simulink model "bh_SIM_7dof_car_MODAL_EXCITE"  (R2021a)
settings: Solver=ode15s  StartTime=0.0  StopTime=5  FixedStep=0.0005  RelTol=1e-5
settings Model: Creator=bhorton  LastModifiedBy=bhorton
settings SolverCC: ZeroCrossAlgorithm=Adaptive
settings ExplorerConfigSet: InternalSimMechanicsExplorerSettings="<ExplorerConfiguration><canonicalview>default</canonicalview><AnimationSetting><BasePlaybackSpeed>1.0</BasePlaybackSpeed><PlaybackSpeedFactor>1.0</PlaybackSpeedFactor></AnimationSetting><TilePanel><TileInfo><Tiles Columns=\"2\" Count=\"3\" Rows=\"2\"><Column Weight=\"0.4994\"/><Column Weight=\"0.5006\"/><Row Weight=\"0.4993\"/><Row Weight=\"0.5007\"/><Tile Height=\"1\" Width=\"2\" X=\"0\" Y=\"0\"/><Tile Height=\"1\" Width=\"1\" X=\"0\" Y=\"1\"/><Tile Height=\"1\" Width=\"1\" X=\"1\" Y=\"1\"/></Tiles></TileInfo><SceneInfo><SceneViewer><BGColor><R>0.60000002384185791</R><G>0.60000002384185791</G><B>0.60000002384185791</B></BGColor><Camera><DoPerspective>off</DoPerspective><Position><X>4.52139190602701735</X><Y>2.25786544378109522</Y><Z>2.39499099381060532</Z></Position><Center><X>2.51193884455935335</X><Y>1.32650226914164038</Y><Z>-0.485736887395236794</Z></Center><Up><X>-0.185673330126828295</X><Y>0.96548958646651295</Y><Z>-0.182634259941381938</Z></Up><ViewLimDist>1</ViewLimDist><YLim>1.8643738979882809</YLim><XLim>3.80619953061108962</XLim></Camera></SceneViewer><SceneViewer><BGColor><R>0.60000002384185791</R><G>0.60000002384185791</G><B>0.60000002384185791</B></BGColor><Camera><DoPerspective>off</DoPerspective><Position><X>1.59253986433018846</X><Y>1.4781034625054259</Y><Z>2.45336125750569334</Z></Position><Center><X>1.41562813270534282</X><Y>1.03964723052633357</Y><Z>-0.792996094118513462</Z></Center><Up><X>-0.0228131350943184333</X><Y>0.990908416802929626</Y><Z>-0.132589857742894418</Z></Up><ViewLimDist>1</ViewLimDist><YLim>1.71081238252217549</YLim><XLim>1.71587395761839479</XLim></Camera></SceneViewer><SceneViewer><BGColor><R>0.60000002384185791</R><G>0.60000002384185791</G><B>0.60000002384185791</B></BGColor><Camera><DoPerspective>off</DoPerspective><Position><X>5.22556337212071131</X><Y>1.49802244333944778</Y><Z>-0.435936726178495881</Z></Position><Center><X>1.55561505094653896</X><Y>1.09424096945505833</Y><Z>-0.658674871233751014</Z></Center><Up><X>-0.109797444713875203</X><Y>0.993927323497863835</Y><Z>0.0072798858972461869</Z></Up><ViewLimDist>1</ViewLimDist><YLim>2.32163445502303123</YLim><XLim>2.33537193700541623</XLim></Camera></SceneViewer></SceneInfo></TilePanel><MechEditorPanel><Cameras/><GfxPanelCameraMap/><VideoCreator><PlaybackSpeedRatio>0.25</PlaybackSpeedRatio><FrameRate>30</FrameRate><VideoFormat>MPEG-4</VideoFormat><FrameSize>[800 600]</FrameSize></VideoCreator></MechEditorPanel></ExplorerConfiguration>"

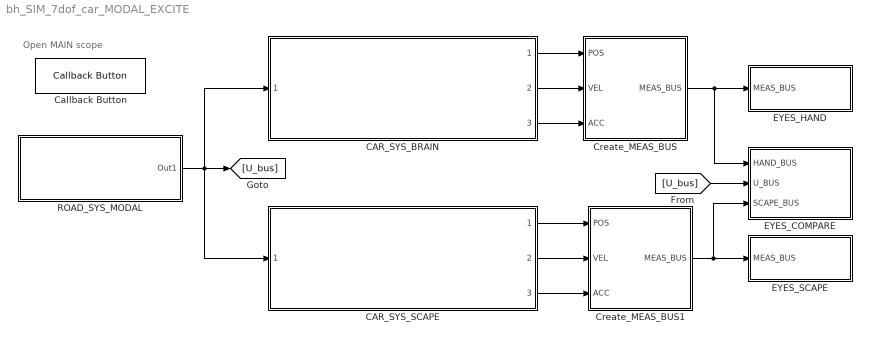
== system bh_SIM_7dof_car_MODAL_EXCITE ==
  note: Open MAIN scope
  CAR_SYS_BRAIN : Subsystem  ReferencedSubsystem=bh_COMPONENT_model_7dof_car_HAND  L_b=OBJ_car_params.L_b  L_f=OBJ_car_params.L_f  L_R=OBJ_car_params.L_R  L_L=OBJ_car_params.L_L  m_c=OBJ_car_params.m_c  I_cZ=OBJ_car_params.I_cZ  I_cX=OBJ_car_params.I_cX  m_bR=OBJ_car_params.m_bR  m_fR=OBJ_car_params.m_fR  m_bL=OBJ_car_params.m_bL  m_fL=OBJ_car_params.m_fL  k_bR=OBJ_car_params.k_bR  k_fR=OBJ_car_params.k_fR  k_bL=OBJ_car_params.k_bL  k_fL=OBJ_car_params.k_fL  k_bRG=OBJ_car_params.k_bRG  k_fRG=OBJ_car_params.k_fRG  k_bLG=OBJ_car_params.k_bLG  k_fLG=OBJ_car_params.k_fLG  c_bR=OBJ_car_params.c_bR  c_fR=OBJ_car_params.c_fR  c_bL=OBJ_car_params.c_bL  c_fL=OBJ_car_params.c_fL  c_bRG=OBJ_car_params.c_bRG  c_fRG=OBJ_car_params.c_fRG  c_bLG=OBJ_car_params.c_bLG  c_fLG=OBJ_car_params.c_fLG  IC_pos=OBJ_car_params.IC_pos  IC_vel=OBJ_car_params.IC_vel
  CAR_SYS_SCAPE : Subsystem  ReferencedSubsystem=bh_COMPONENT_model_7dof_car_SCAPE  L_b=OBJ_car_params.L_b  L_f=OBJ_car_params.L_f  L_R=OBJ_car_params.L_R  L_L=OBJ_car_params.L_L  m_c=OBJ_car_params.m_c  I_cZ=OBJ_car_params.I_cZ  I_cX=OBJ_car_params.I_cX  m_bR=OBJ_car_params.m_bR  m_fR=OBJ_car_params.m_fR  m_bL=OBJ_car_params.m_bL  m_fL=OBJ_car_params.m_fL  k_bR=OBJ_car_params.k_bR  k_fR=OBJ_car_params.k_fR  k_bL=OBJ_car_params.k_bL  k_fL=OBJ_car_params.k_fL  k_bRG=OBJ_car_params.k_bRG  k_fRG=OBJ_car_params.k_fRG  k_bLG=OBJ_car_params.k_bLG  k_fLG=OBJ_car_params.k_fLG  c_bR=OBJ_car_params.c_bR  c_fR=OBJ_car_params.c_fR  c_bL=OBJ_car_params.c_bL  c_fL=OBJ_car_params.c_fL  c_bRG=OBJ_car_params.c_bRG  c_fRG=OBJ_car_params.c_fRG  c_bLG=OBJ_car_params.c_bLG  c_fLG=OBJ_car_params.c_fLG  IC_pos=OBJ_car_params.IC_pos  IC_vel=OBJ_car_params.IC_vel
  Callback Button : CallbackButton  ButtonText=CLICK me to open SCOPE
      settings: ClickFcn=open_system([bdroot,'/EYES_COMPARE/COMPARE_POS'])
  Create_MEAS_BUS : Subsystem
  Create_MEAS_BUS1 : Subsystem
  EYES_COMPARE : Subsystem
  EYES_HAND : Subsystem
  EYES_SCAPE : Subsystem
  ROAD_SYS_MODAL : Subsystem  mask(ROAD_MODAL_EXCITATION){m_AMP=0.03, m_excite_type=bh_excite_mode_ENUM_CLS.MODAL_Y_BOUNCE, f_str=3, m_mode_table={'1', 'BOUNCE','0.9162';  '2', 'ROLL','1.1836';  '3', 'PITCH','1.6742';  '4', 'FRONT_OUT_PHASE','5.6358';  '5', 'FRONT_IN_PHASE','5.6435';  '6', 'BACK_OUT_PHASE','6.2992';  '7', 'BACK_IN_PHASE','6.3188'}}
      mask prompts: m_AMP "Amplitude (m)"; m_excite_type "Excitation Type"; f_str "f (Hz)"; m_mode_table "The Modes (the table is NOT editable)"
      mask help:
      | ATTENTION:
      |
      | The MODAL frequencies are HARD CODED in the function bh_road_modal_callback().
      |
      | So? - So if you configure the car with different parameters(m,ck, etc) then you need to update the above file with your UNdamped modal frequencies.
      mask init:
      | % ATTENTION:
      | %   there is a CALLBACK attached to the "m_excite_type"
      | %   parameter which ENABLES or DISABLES the "f_str"
      | %   parameter.  See the file:
      | %
      | %    --->  bh_road_modal_callback.m
      | 
      | f_hz            = str2num(f_str);
      | excite_type_str = string(m_excite_type);
      | amp_str         = num2str(m_AMP);
      | 
      | str0 = sprintf('%s',excite_type_str);
      | str1 = sprintf('Amp = %s', amp_str);
      | 
      | tf_sine_excite = m_excite_type.isSineMember();
      | 
      | f_hz_modal = 0;
      | 
      | if(tf_sine_excite)
      |     str2 = sprintf('Freq = %d (Hz)',f_hz);
      | else
      |     f_hz_modal = bh_road_modal_callback("GET_FHZ_MODAL", gcb);
      |     str2       = sprintf('Freq = %.4f (Hz)',f_hz_modal);
      | end
      | 
      | str  = char(str0,str1,str2);
      | 
      | bh_road_modal_callback("POPULATE_TABLE", gcb);
      mask Callback m_excite_type: bh_road_modal_callback("M_EXCITE_CBACK", gcb)
      mask TypeOptions f_str: 0 | 1 | 2 | 3 | 5 | 10 | 20 | 50 | 100
      mask DialogControl Container3 Prompt: Edit the following file to define your MODAL frequencies
      mask DialogControl Control2 Prompt: CLICK ME TO EDIT FILE
      mask DialogControl Control2 Callback: bh_road_modal_callback("EDIT_THIS_FILE",gcb)
      mask Display: disp(str)
  wires:
  CAR_SYS_BRAIN/1 -> Create_MEAS_BUS/1(POS)
  CAR_SYS_BRAIN/2 -> Create_MEAS_BUS/2(VEL)
  CAR_SYS_BRAIN/3 -> Create_MEAS_BUS/3(ACC)
  Create_MEAS_BUS/1(MEAS_BUS) -> EYES_COMPARE/1(HAND_BUS), EYES_HAND/1(MEAS_BUS)
  CAR_SYS_SCAPE/1 -> Create_MEAS_BUS1/1(POS)
  CAR_SYS_SCAPE/2 -> Create_MEAS_BUS1/2(VEL)
  CAR_SYS_SCAPE/3 -> Create_MEAS_BUS1/3(ACC)
  Create_MEAS_BUS1/1(MEAS_BUS) -> EYES_COMPARE/3(SCAPE_BUS), EYES_SCAPE/1(MEAS_BUS)
  ROAD_SYS_MODAL/1(Out1) -> [U_bus], CAR_SYS_BRAIN/1, CAR_SYS_SCAPE/1
  [U_bus] -> EYES_COMPARE/2(U_BUS)

== system bh_SIM_7dof_car_MODAL_EXCITE/Create_MEAS_BUS ==
  POS : Inport
  VEL : Inport  Port=2
  ACC : Inport  Port=3
  Bus Creator : BusCreator  Inputs=3
  MEAS_BUS : Outport
  wires:
  POS/1 -> Bus Creator/1  "POS"
  VEL/1 -> Bus Creator/2  "VEL"
  ACC/1 -> Bus Creator/3  "ACC"
  Bus Creator/1 -> MEAS_BUS/1

== system bh_SIM_7dof_car_MODAL_EXCITE/Create_MEAS_BUS1 ==
  POS : Inport
  VEL : Inport  Port=2
  ACC : Inport  Port=3
  Bus Creator : BusCreator  Inputs=3
  MEAS_BUS : Outport
  wires:
  POS/1 -> Bus Creator/1  "POS"
  VEL/1 -> Bus Creator/2  "VEL"
  ACC/1 -> Bus Creator/3  "ACC"
  Bus Creator/1 -> MEAS_BUS/1

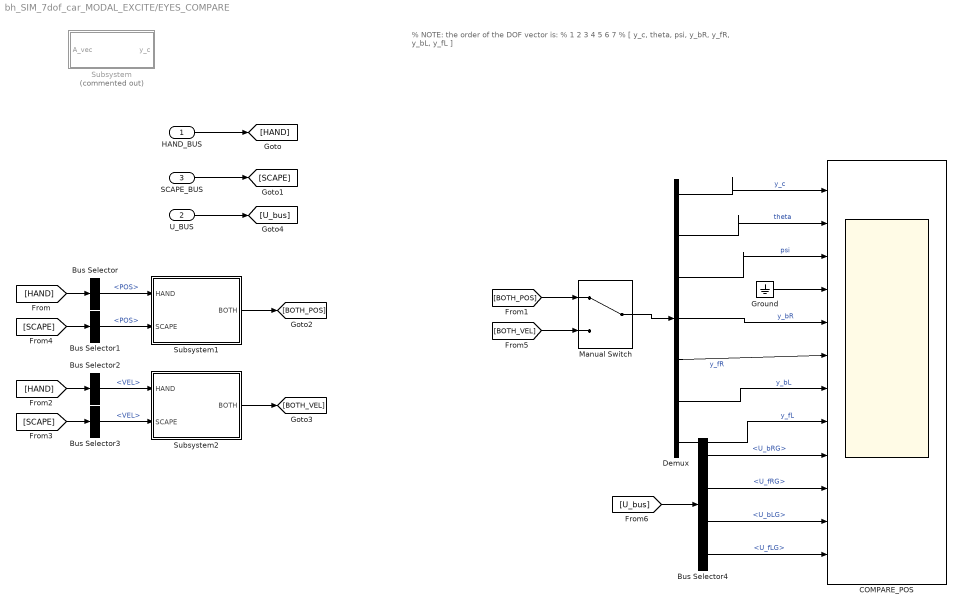
== system bh_SIM_7dof_car_MODAL_EXCITE/EYES_COMPARE ==
  note: % NOTE:  the order of the DOF vector is:
      | %          1      2    3     4     5     6     7
      | %      [ y_c, theta, psi, y_bR, y_fR, y_bL, y_fL ]
  HAND_BUS : Inport
  U_BUS : Inport  Port=2
  SCAPE_BUS : Inport  Port=3
  Bus Selector : BusSelector  OutputSignals=POS
  Bus Selector1 : BusSelector  OutputSignals=POS
  Bus Selector2 : BusSelector  OutputSignals=VEL
  Bus Selector3 : BusSelector  OutputSignals=VEL
  Bus Selector4 : BusSelector  OutputSignals=U_bRG,U_fRG,U_bLG,U_fLG
  COMPARE_POS : Scope  NumInputPorts=12
  Demux : Demux  Outputs=7
  Ground : Ground
  Manual Switch : ManualSwitch
  Subsystem : Subsystem  Commented=on
  Subsystem1 : Subsystem
  Subsystem2 : Subsystem
  wires:
  HAND_BUS/1 -> [HAND]
  Demux/1 -> COMPARE_POS/1  "y_c"
  Demux/2 -> COMPARE_POS/2  "theta"
  Demux/3 -> COMPARE_POS/3  "psi"
  Ground/1 -> COMPARE_POS/4
  Demux/4 -> COMPARE_POS/5  "y_bR"
  Demux/5 -> COMPARE_POS/6  "y_fR"
  Demux/6 -> COMPARE_POS/7  "y_bL"
  Demux/7 -> COMPARE_POS/8  "y_fL"
  SCAPE_BUS/1 -> [SCAPE]
  [HAND] -> Bus Selector/1
  [SCAPE] -> Bus Selector1/1
  Bus Selector/1 -> Subsystem1/1(HAND)  "<POS>"
  Bus Selector1/1 -> Subsystem1/2(SCAPE)  "<POS>"
  Subsystem1/1(BOTH) -> [BOTH_POS]
  [HAND] -> Bus Selector2/1
  Subsystem2/1(BOTH) -> [BOTH_VEL]
  Bus Selector2/1 -> Subsystem2/1(HAND)  "<VEL>"
  Bus Selector3/1 -> Subsystem2/2(SCAPE)  "<VEL>"
  [SCAPE] -> Bus Selector3/1
  Manual Switch/1 -> Demux/1
  [BOTH_VEL] -> Manual Switch/2
  [BOTH_POS] -> Manual Switch/1
  U_BUS/1 -> [U_bus]
  [U_bus] -> Bus Selector4/1
  Bus Selector4/4 -> COMPARE_POS/12  "<U_fLG>"
  Bus Selector4/3 -> COMPARE_POS/11  "<U_bLG>"
  Bus Selector4/2 -> COMPARE_POS/10  "<U_fRG>"
  Bus Selector4/1 -> COMPARE_POS/9  "<U_bRG>"

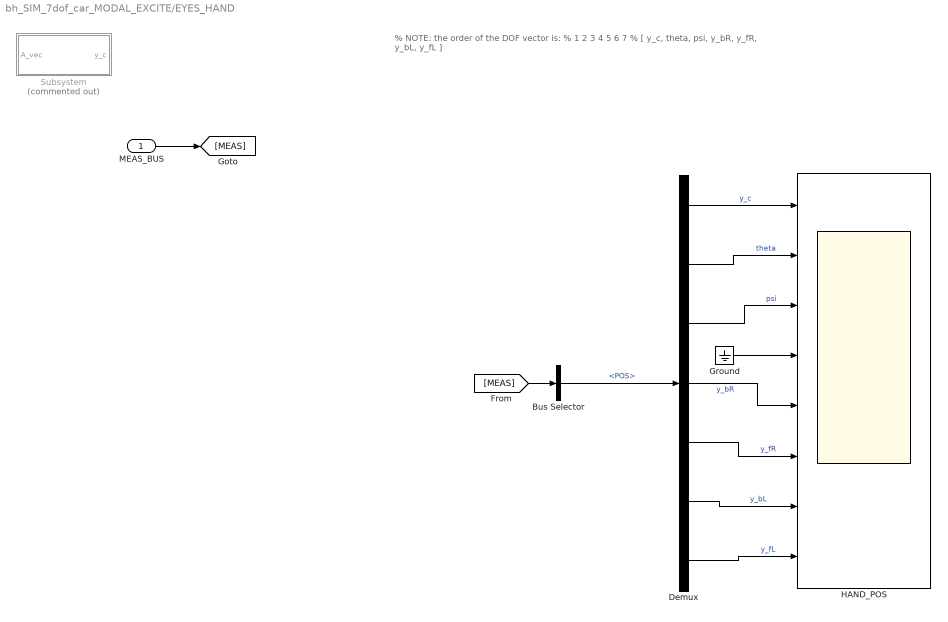
== system bh_SIM_7dof_car_MODAL_EXCITE/EYES_HAND ==
  note: % NOTE:  the order of the DOF vector is:
      | %          1      2    3     4     5     6     7
      | %      [ y_c, theta, psi, y_bR, y_fR, y_bL, y_fL ]
  MEAS_BUS : Inport
  Bus Selector : BusSelector  OutputSignals=POS
  Demux : Demux  Outputs=7
  Ground : Ground
  HAND_POS : Scope  NumInputPorts=8
  Subsystem : Subsystem  Commented=on
  wires:
  MEAS_BUS/1 -> [MEAS]
  Demux/1 -> HAND_POS/1  "y_c"
  Demux/2 -> HAND_POS/2  "theta"
  Demux/3 -> HAND_POS/3  "psi"
  Ground/1 -> HAND_POS/4
  Demux/4 -> HAND_POS/5  "y_bR"
  Demux/5 -> HAND_POS/6  "y_fR"
  Demux/6 -> HAND_POS/7  "y_bL"
  Demux/7 -> HAND_POS/8  "y_fL"
  [MEAS] -> Bus Selector/1
  Bus Selector/1 -> Demux/1  "<POS>"

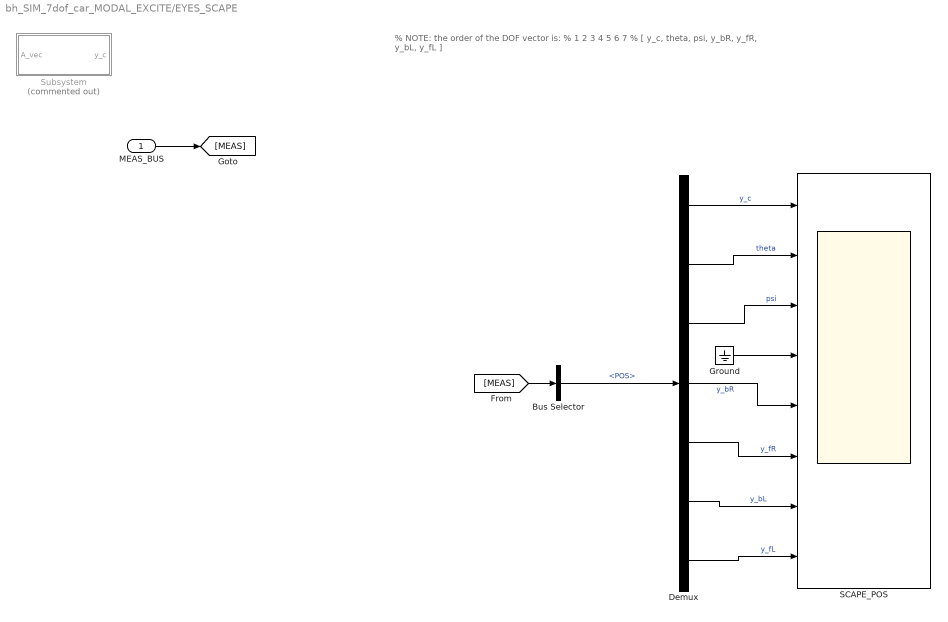
== system bh_SIM_7dof_car_MODAL_EXCITE/EYES_SCAPE ==
  note: % NOTE:  the order of the DOF vector is:
      | %          1      2    3     4     5     6     7
      | %      [ y_c, theta, psi, y_bR, y_fR, y_bL, y_fL ]
  MEAS_BUS : Inport
  Bus Selector : BusSelector  OutputSignals=POS
  Demux : Demux  Outputs=7
  Ground : Ground
  SCAPE_POS : Scope  NumInputPorts=8
  Subsystem : Subsystem  Commented=on
  wires:
  MEAS_BUS/1 -> [MEAS]
  Demux/1 -> SCAPE_POS/1  "y_c"
  Demux/2 -> SCAPE_POS/2  "theta"
  Demux/3 -> SCAPE_POS/3  "psi"
  Ground/1 -> SCAPE_POS/4
  Demux/4 -> SCAPE_POS/5  "y_bR"
  Demux/5 -> SCAPE_POS/6  "y_fR"
  Demux/6 -> SCAPE_POS/7  "y_bL"
  Demux/7 -> SCAPE_POS/8  "y_fL"
  [MEAS] -> Bus Selector/1
  Bus Selector/1 -> Demux/1  "<POS>"

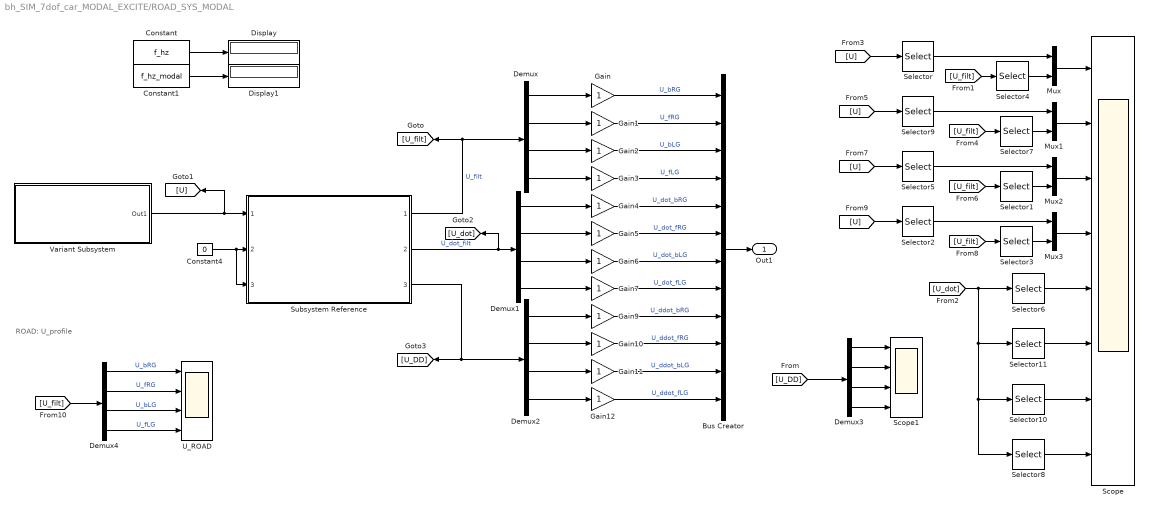
== system bh_SIM_7dof_car_MODAL_EXCITE/ROAD_SYS_MODAL ==
  note: ROAD: U_profile
  Bus Creator : BusCreator  Inputs=12
  Constant : Constant  Value=f_hz
  Constant1 : Constant  Value=f_hz_modal
  Constant4 : Constant  Value=0
  Demux{,1..4} (5 alike) : Demux
  Display : Display
  Display1 : Display
  Gain{,1..7,9..12} (12 alike) : Gain
  Mux{,1..3} (4 alike) : Mux  Inputs=2
  Scope : Scope  NumInputPorts=8
  Scope1 : Scope  NumInputPorts=4
  Selector : Selector  InputPortWidth=4  IndexOptions=Index vector (dialog)  Indices=1  OutputSizes=1
  Selector1 : Selector  InputPortWidth=4  IndexOptions=Index vector (dialog)  Indices=3  OutputSizes=1
  Selector10 : Selector  InputPortWidth=4  IndexOptions=Index vector (dialog)  Indices=3  OutputSizes=1
  Selector11 : Selector  InputPortWidth=4  IndexOptions=Index vector (dialog)  Indices=2  OutputSizes=1
  Selector2 : Selector  InputPortWidth=4  IndexOptions=Index vector (dialog)  Indices=4  OutputSizes=1
  Selector3 : Selector  InputPortWidth=4  IndexOptions=Index vector (dialog)  Indices=4  OutputSizes=1
  Selector4 : Selector  InputPortWidth=4  IndexOptions=Index vector (dialog)  Indices=1  OutputSizes=1
  Selector5 : Selector  InputPortWidth=4  IndexOptions=Index vector (dialog)  Indices=3  OutputSizes=1
  Selector6 : Selector  InputPortWidth=4  IndexOptions=Index vector (dialog)  Indices=1  OutputSizes=1
  Selector7 : Selector  InputPortWidth=4  IndexOptions=Index vector (dialog)  Indices=2  OutputSizes=1
  Selector8 : Selector  InputPortWidth=4  IndexOptions=Index vector (dialog)  Indices=4  OutputSizes=1
  Selector9 : Selector  InputPortWidth=4  IndexOptions=Index vector (dialog)  Indices=2  OutputSizes=1
  Subsystem Reference : Subsystem  ReferencedSubsystem=bh_COMPONENT_deriv_est  wn=2*pi*5000  p=1
  U_ROAD : Scope  NumInputPorts=4
  Variant Subsystem : Subsystem  Variant=on
  Out1 : Outport
  wires:
  Gain/1 -> Bus Creator/1  "U_bRG"
  Gain1/1 -> Bus Creator/2  "U_fRG"
  Gain2/1 -> Bus Creator/3  "U_bLG"
  Gain3/1 -> Bus Creator/4  "U_fLG"
  Bus Creator/1 -> Out1/1
  Gain4/1 -> Bus Creator/5  "U_dot_bRG"
  Gain6/1 -> Bus Creator/7  "U_dot_bLG"
  Gain5/1 -> Bus Creator/6  "U_dot_fRG"
  Gain7/1 -> Bus Creator/8  "U_dot_fLG"
  Variant Subsystem/1(Out1) -> Subsystem Reference/1, [U]
  Demux/4 -> Gain3/1
  Demux/3 -> Gain2/1
  Demux/2 -> Gain1/1
  Demux/1 -> Gain/1
  Demux1/1 -> Gain4/1
  Demux1/2 -> Gain5/1
  Demux1/3 -> Gain6/1
  Demux1/4 -> Gain7/1
  Mux3/1 -> Scope/4
  Mux2/1 -> Scope/3
  Mux1/1 -> Scope/2
  Mux/1 -> Scope/1
  Selector4/1 -> Mux/2
  Selector/1 -> Mux/1
  [U_filt] -> Selector4/1
  [U] -> Selector/1
  Selector7/1 -> Mux1/2
  [U_filt] -> Selector7/1
  [U] -> Selector9/1
  Selector9/1 -> Mux1/1
  Selector1/1 -> Mux2/2
  [U_filt] -> Selector1/1
  [U] -> Selector5/1
  Selector5/1 -> Mux2/1
  Selector3/1 -> Mux3/2
  [U_filt] -> Selector3/1
  [U] -> Selector2/1
  Selector2/1 -> Mux3/1
  [U_dot] -> Selector11/1, Selector10/1, Selector8/1, Selector6/1
  Selector8/1 -> Scope/8
  Selector10/1 -> Scope/7
  Selector11/1 -> Scope/6
  Selector6/1 -> Scope/5
  Constant/1 -> Display/1
  Demux2/2 -> Gain10/1
  Demux2/4 -> Gain12/1
  Demux2/3 -> Gain11/1
  Demux2/1 -> Gain9/1
  Gain9/1 -> Bus Creator/9  "U_ddot_bRG"
  Gain10/1 -> Bus Creator/10  "U_ddot_fRG"
  Gain11/1 -> Bus Creator/11  "U_ddot_bLG"
  Gain12/1 -> Bus Creator/12  "U_ddot_fLG"
  Demux3/4 -> Scope1/4
  Demux3/3 -> Scope1/3
  Demux3/2 -> Scope1/2
  Demux3/1 -> Scope1/1
  [U_DD] -> Demux3/1
  Constant4/1 -> Subsystem Reference/3, Subsystem Reference/2
  Subsystem Reference/2 -> [U_dot], Demux1/1  "U_dot_filt"
  Subsystem Reference/1 -> [U_filt], Demux/1  "U_filt"
  Subsystem Reference/3 -> [U_DD], Demux2/1
  Constant1/1 -> Display1/1
  [U_filt] -> Demux4/1
  Demux4/1 -> U_ROAD/1  "U_bRG"
  Demux4/2 -> U_ROAD/2  "U_fRG"
  Demux4/3 -> U_ROAD/3  "U_bLG"
  Demux4/4 -> U_ROAD/4  "U_fLG"

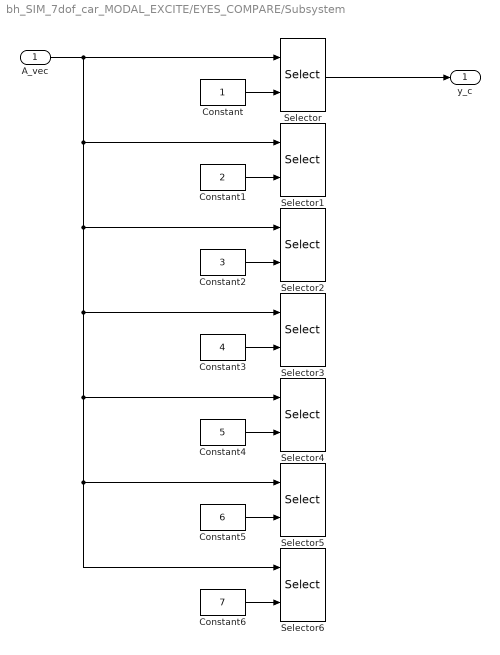
== system bh_SIM_7dof_car_MODAL_EXCITE/EYES_COMPARE/Subsystem ==
  A_vec : Inport
  Constant : Constant
  Constant1 : Constant  Value=2
  Constant2 : Constant  Value=3
  Constant3 : Constant  Value=4
  Constant4 : Constant  Value=5
  Constant5 : Constant  Value=6
  Constant6 : Constant  Value=7
  Selector{,1..6} (7 alike) : Selector  InputPortWidth=7  IndexOptions=Index vector (port)  Indices=1  OutputSizes=1
  y_c : Outport
  wires:
  Constant/1 -> Selector/2
  Constant1/1 -> Selector1/2
  Constant2/1 -> Selector2/2
  Constant3/1 -> Selector3/2
  Constant4/1 -> Selector4/2
  Constant5/1 -> Selector5/2
  Constant6/1 -> Selector6/2
  A_vec/1 -> Selector1/1, Selector2/1, Selector3/1, Selector4/1, Selector5/1, Selector6/1, Selector/1
  Selector/1 -> y_c/1

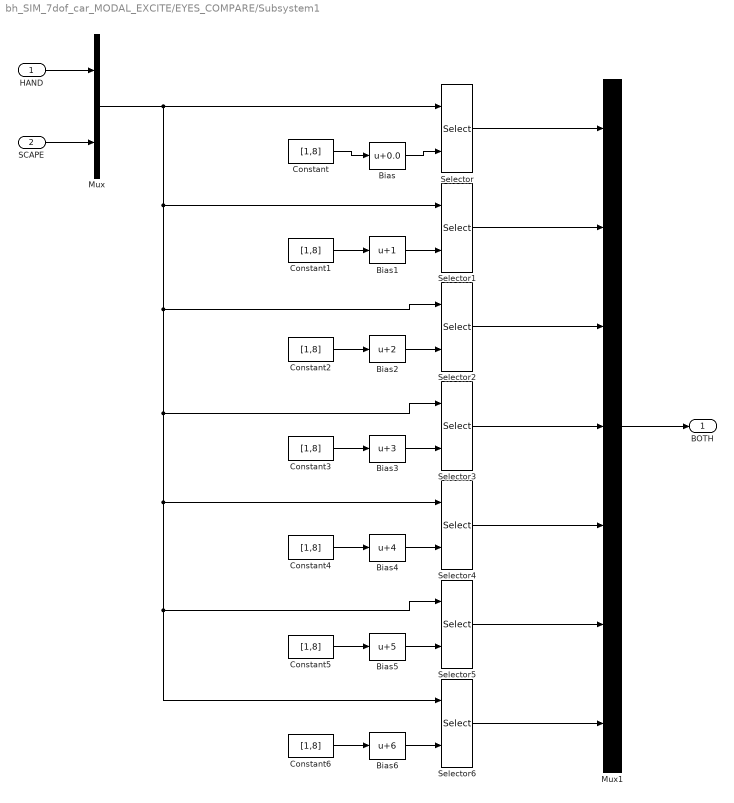
== system bh_SIM_7dof_car_MODAL_EXCITE/EYES_COMPARE/Subsystem1 ==
  HAND : Inport
  SCAPE : Inport  Port=2
  Bias : Bias  Bias=0.0
  Bias1 : Bias  Bias=1
  Bias2 : Bias  Bias=2
  Bias3 : Bias  Bias=3
  Bias4 : Bias  Bias=4
  Bias5 : Bias  Bias=5
  Bias6 : Bias  Bias=6
  Constant{,1..6} (7 alike) : Constant  Value=[1,8]
  Mux : Mux  Inputs=2
  Mux1 : Mux  Inputs=7
  Selector{,1..6} (7 alike) : Selector  InputPortWidth=14  IndexOptions=Index vector (port)  Indices=[1 3]  OutputSizes=1
  BOTH : Outport
  wires:
  SCAPE/1 -> Mux/2
  HAND/1 -> Mux/1
  Constant/1 -> Bias/1
  Bias/1 -> Selector/2
  Selector/1 -> Mux1/1
  Selector1/1 -> Mux1/2
  Bias1/1 -> Selector1/2
  Constant1/1 -> Bias1/1
  Constant2/1 -> Bias2/1
  Bias2/1 -> Selector2/2
  Selector2/1 -> Mux1/3
  Bias3/1 -> Selector3/2
  Constant3/1 -> Bias3/1
  Selector3/1 -> Mux1/4
  Constant4/1 -> Bias4/1
  Bias4/1 -> Selector4/2
  Selector4/1 -> Mux1/5
  Constant5/1 -> Bias5/1
  Bias5/1 -> Selector5/2
  Constant6/1 -> Bias6/1
  Bias6/1 -> Selector6/2
  Mux/1 -> Selector1/1, Selector2/1, Selector3/1, Selector4/1, Selector5/1, Selector6/1, Selector/1
  Selector5/1 -> Mux1/6
  Selector6/1 -> Mux1/7
  Mux1/1 -> BOTH/1

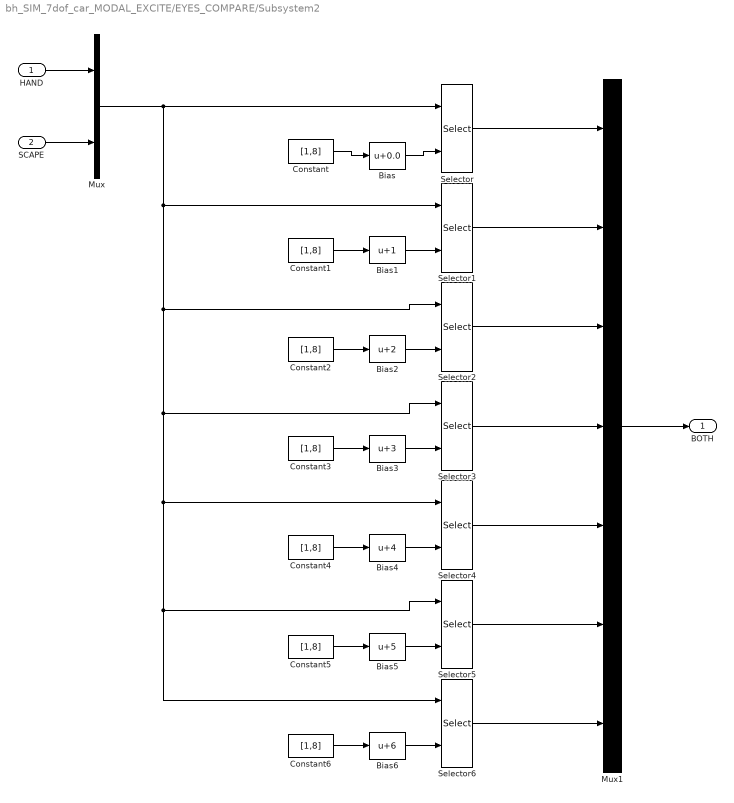
== system bh_SIM_7dof_car_MODAL_EXCITE/EYES_COMPARE/Subsystem2 ==
  HAND : Inport
  SCAPE : Inport  Port=2
  Bias : Bias  Bias=0.0
  Bias1 : Bias  Bias=1
  Bias2 : Bias  Bias=2
  Bias3 : Bias  Bias=3
  Bias4 : Bias  Bias=4
  Bias5 : Bias  Bias=5
  Bias6 : Bias  Bias=6
  Constant{,1..6} (7 alike) : Constant  Value=[1,8]
  Mux : Mux  Inputs=2
  Mux1 : Mux  Inputs=7
  Selector{,1..6} (7 alike) : Selector  InputPortWidth=14  IndexOptions=Index vector (port)  Indices=[1 3]  OutputSizes=1
  BOTH : Outport
  wires:
  SCAPE/1 -> Mux/2
  HAND/1 -> Mux/1
  Constant/1 -> Bias/1
  Bias/1 -> Selector/2
  Selector/1 -> Mux1/1
  Selector1/1 -> Mux1/2
  Bias1/1 -> Selector1/2
  Constant1/1 -> Bias1/1
  Constant2/1 -> Bias2/1
  Bias2/1 -> Selector2/2
  Selector2/1 -> Mux1/3
  Bias3/1 -> Selector3/2
  Constant3/1 -> Bias3/1
  Selector3/1 -> Mux1/4
  Constant4/1 -> Bias4/1
  Bias4/1 -> Selector4/2
  Selector4/1 -> Mux1/5
  Constant5/1 -> Bias5/1
  Bias5/1 -> Selector5/2
  Constant6/1 -> Bias6/1
  Bias6/1 -> Selector6/2
  Mux/1 -> Selector1/1, Selector2/1, Selector3/1, Selector4/1, Selector5/1, Selector6/1, Selector/1
  Selector5/1 -> Mux1/6
  Selector6/1 -> Mux1/7
  Mux1/1 -> BOTH/1

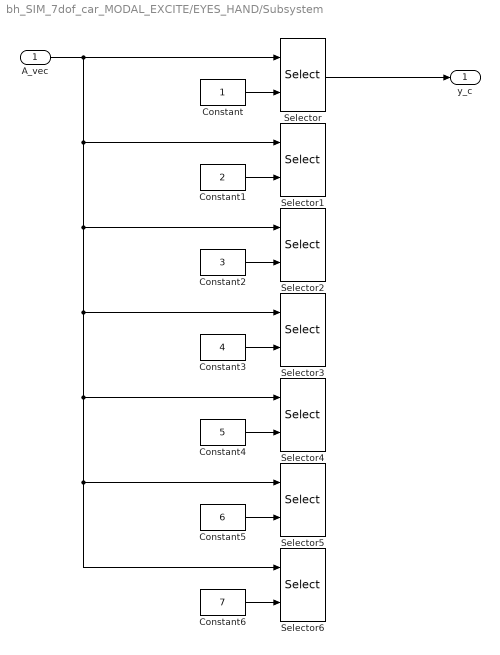
== system bh_SIM_7dof_car_MODAL_EXCITE/EYES_HAND/Subsystem ==
  A_vec : Inport
  Constant : Constant
  Constant1 : Constant  Value=2
  Constant2 : Constant  Value=3
  Constant3 : Constant  Value=4
  Constant4 : Constant  Value=5
  Constant5 : Constant  Value=6
  Constant6 : Constant  Value=7
  Selector{,1..6} (7 alike) : Selector  InputPortWidth=7  IndexOptions=Index vector (port)  Indices=1  OutputSizes=1
  y_c : Outport
  wires:
  Constant/1 -> Selector/2
  Constant1/1 -> Selector1/2
  Constant2/1 -> Selector2/2
  Constant3/1 -> Selector3/2
  Constant4/1 -> Selector4/2
  Constant5/1 -> Selector5/2
  Constant6/1 -> Selector6/2
  A_vec/1 -> Selector1/1, Selector2/1, Selector3/1, Selector4/1, Selector5/1, Selector6/1, Selector/1
  Selector/1 -> y_c/1

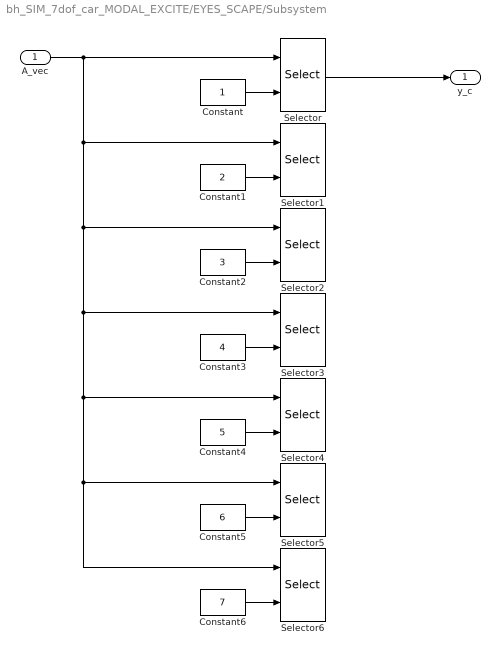
== system bh_SIM_7dof_car_MODAL_EXCITE/EYES_SCAPE/Subsystem ==
  A_vec : Inport
  Constant : Constant
  Constant1 : Constant  Value=2
  Constant2 : Constant  Value=3
  Constant3 : Constant  Value=4
  Constant4 : Constant  Value=5
  Constant5 : Constant  Value=6
  Constant6 : Constant  Value=7
  Selector{,1..6} (7 alike) : Selector  InputPortWidth=7  IndexOptions=Index vector (port)  Indices=1  OutputSizes=1
  y_c : Outport
  wires:
  Constant/1 -> Selector/2
  Constant1/1 -> Selector1/2
  Constant2/1 -> Selector2/2
  Constant3/1 -> Selector3/2
  Constant4/1 -> Selector4/2
  Constant5/1 -> Selector5/2
  Constant6/1 -> Selector6/2
  A_vec/1 -> Selector1/1, Selector2/1, Selector3/1, Selector4/1, Selector5/1, Selector6/1, Selector/1
  Selector/1 -> y_c/1

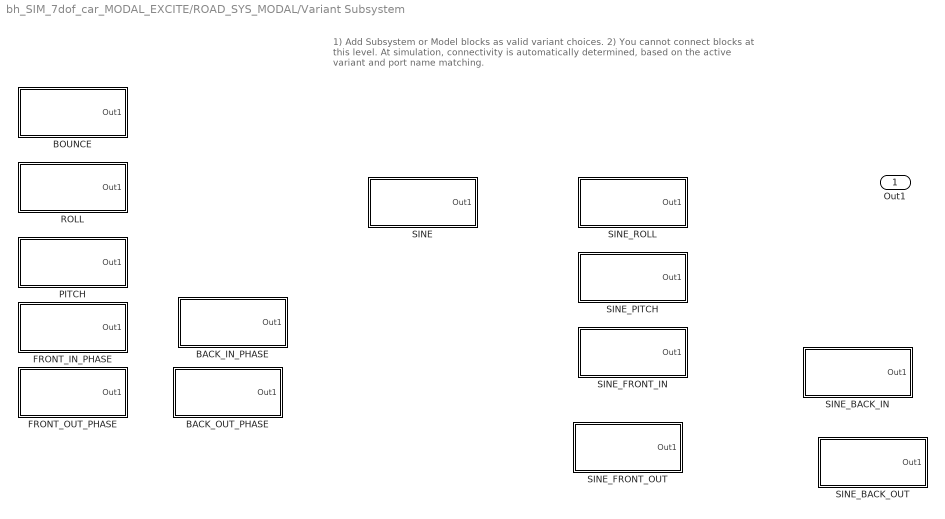
== system bh_SIM_7dof_car_MODAL_EXCITE/ROAD_SYS_MODAL/Variant Subsystem ==
  note: 1) Add Subsystem or Model blocks as valid variant choices.
      | 2) You cannot connect blocks at this level. At simulation, connectivity is automatically
      | determined, based on the active variant and port name matching.
  BACK_IN_PHASE : Subsystem  VariantControl=m_excite_type==bh_excite_mode_ENUM_CLS.MODAL_BACK_IN_PHASE
  BACK_OUT_PHASE : Subsystem  VariantControl=m_excite_type==bh_excite_mode_ENUM_CLS.MODAL_BACK_OUT_PHASE
  BOUNCE : Subsystem  VariantControl=m_excite_type==bh_excite_mode_ENUM_CLS.MODAL_Y_BOUNCE
  FRONT_IN_PHASE : Subsystem  VariantControl=m_excite_type==bh_excite_mode_ENUM_CLS.MODAL_FRONT_IN_PHASE
  FRONT_OUT_PHASE : Subsystem  VariantControl=m_excite_type==bh_excite_mode_ENUM_CLS.MODAL_FRONT_OUT_PHASE
  PITCH : Subsystem  VariantControl=m_excite_type==bh_excite_mode_ENUM_CLS.MODAL_PITCH
  ROLL : Subsystem  VariantControl=m_excite_type==bh_excite_mode_ENUM_CLS.MODAL_ROLL
  SINE : Subsystem  VariantControl=m_excite_type==bh_excite_mode_ENUM_CLS.SINE
  SINE_BACK_IN : Subsystem  VariantControl=m_excite_type==bh_excite_mode_ENUM_CLS.SINE_BACK_IN_PHASE
  SINE_BACK_OUT : Subsystem  VariantControl=m_excite_type==bh_excite_mode_ENUM_CLS.SINE_BACK_OUT_PHASE
  SINE_FRONT_IN : Subsystem  VariantControl=m_excite_type==bh_excite_mode_ENUM_CLS.SINE_FRONT_IN_PHASE
  SINE_FRONT_OUT : Subsystem  VariantControl=m_excite_type==bh_excite_mode_ENUM_CLS.SINE_FRONT_OUT_PHASE
  SINE_PITCH : Subsystem  VariantControl=m_excite_type==bh_excite_mode_ENUM_CLS.SINE_PITCH
  SINE_ROLL : Subsystem  VariantControl=m_excite_type==bh_excite_mode_ENUM_CLS.SINE_ROLL
  Out1 : Outport

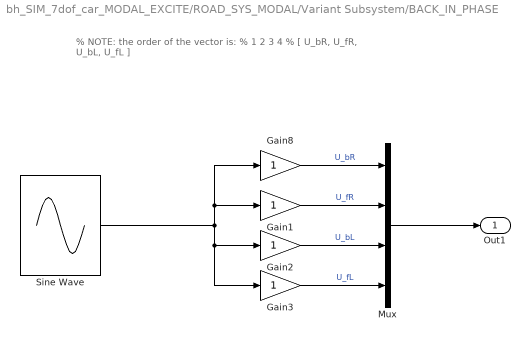
== system bh_SIM_7dof_car_MODAL_EXCITE/ROAD_SYS_MODAL/Variant Subsystem/BACK_IN_PHASE ==
  note: % NOTE:  the order of the vector is:
      | %       1      2     3     4
      | %     [ U_bR,  U_fR, U_bL, U_fL ]
  Gain{1..3,8} (4 alike) : Gain
  Mux : Mux
  Sine Wave : Sin  Amplitude=m_AMP  Frequency=2*pi*f_hz_modal  SampleTime=0
      settings: AttributesFormatString=|
      | Amp =%<Amplitude>
      | w_radpsec = %<Frequency>
  Out1 : Outport
  wires:
  Gain8/1 -> Mux/1  "U_bR"
  Gain1/1 -> Mux/2  "U_fR"
  Gain2/1 -> Mux/3  "U_bL"
  Gain3/1 -> Mux/4  "U_fL"
  Sine Wave/1 -> Gain8/1, Gain1/1, Gain2/1, Gain3/1
  Mux/1 -> Out1/1

== system bh_SIM_7dof_car_MODAL_EXCITE/ROAD_SYS_MODAL/Variant Subsystem/BACK_OUT_PHASE ==
  note: % NOTE:  the order of the vector is:
      | %       1      2     3     4
      | %     [ U_bR,  U_fR, U_bL, U_fL ]
  Gain1 : Gain
  Gain2 : Gain  Gain=-1
  Gain3 : Gain
  Gain8 : Gain
  Mux : Mux
  Sine Wave : Sin  Amplitude=m_AMP  Frequency=2*pi*f_hz_modal  SampleTime=0
      settings: AttributesFormatString=|
      | Amp =%<Amplitude>
      | w_radpsec = %<Frequency>
  Out1 : Outport
  wires:
  Gain8/1 -> Mux/1  "U_bR"
  Gain1/1 -> Mux/2  "U_fR"
  Gain2/1 -> Mux/3  "U_bL"
  Gain3/1 -> Mux/4  "U_fL"
  Sine Wave/1 -> Gain8/1, Gain1/1, Gain2/1, Gain3/1
  Mux/1 -> Out1/1

== system bh_SIM_7dof_car_MODAL_EXCITE/ROAD_SYS_MODAL/Variant Subsystem/BOUNCE ==
  note: % NOTE:  the order of the vector is:
      | %       1      2     3     4
      | %     [ U_bR,  U_fR, U_bL, U_fL ]
  Gain{1..3,8} (4 alike) : Gain
  Mux : Mux
  Sine Wave : Sin  Amplitude=m_AMP  Frequency=2*pi*f_hz_modal  SampleTime=0
      settings: AttributesFormatString=|
      | Amp =%<Amplitude>
      | w_radpsec = %<Frequency>
  Out1 : Outport
  wires:
  Gain8/1 -> Mux/1  "U_bR"
  Gain1/1 -> Mux/2  "U_fR"
  Gain2/1 -> Mux/3  "U_bL"
  Gain3/1 -> Mux/4  "U_fL"
  Sine Wave/1 -> Gain8/1, Gain1/1, Gain2/1, Gain3/1
  Mux/1 -> Out1/1

== system bh_SIM_7dof_car_MODAL_EXCITE/ROAD_SYS_MODAL/Variant Subsystem/FRONT_IN_PHASE ==
  note: % NOTE:  the order of the vector is:
      | %       1      2     3     4
      | %     [ U_bR,  U_fR, U_bL, U_fL ]
  Gain{1..3,8} (4 alike) : Gain
  Mux : Mux
  Sine Wave : Sin  Amplitude=m_AMP  Frequency=2*pi*f_hz_modal  SampleTime=0
      settings: AttributesFormatString=|
      | Amp =%<Amplitude>
      | w_radpsec = %<Frequency>
  Out1 : Outport
  wires:
  Gain8/1 -> Mux/1  "U_bR"
  Gain1/1 -> Mux/2  "U_fR"
  Gain2/1 -> Mux/3  "U_bL"
  Gain3/1 -> Mux/4  "U_fL"
  Sine Wave/1 -> Gain8/1, Gain1/1, Gain2/1, Gain3/1
  Mux/1 -> Out1/1

== system bh_SIM_7dof_car_MODAL_EXCITE/ROAD_SYS_MODAL/Variant Subsystem/FRONT_OUT_PHASE ==
  note: % NOTE:  the order of the vector is:
      | %       1      2     3     4
      | %     [ U_bR,  U_fR, U_bL, U_fL ]
  Gain1 : Gain  Gain=-1
  Gain2 : Gain
  Gain3 : Gain
  Gain8 : Gain
  Mux : Mux
  Sine Wave : Sin  Amplitude=m_AMP  Frequency=2*pi*f_hz_modal  SampleTime=0
      settings: AttributesFormatString=|
      | Amp =%<Amplitude>
      | w_radpsec = %<Frequency>
  Out1 : Outport
  wires:
  Gain8/1 -> Mux/1  "U_bR"
  Gain1/1 -> Mux/2  "U_fR"
  Gain2/1 -> Mux/3  "U_bL"
  Gain3/1 -> Mux/4  "U_fL"
  Sine Wave/1 -> Gain8/1, Gain1/1, Gain2/1, Gain3/1
  Mux/1 -> Out1/1

== system bh_SIM_7dof_car_MODAL_EXCITE/ROAD_SYS_MODAL/Variant Subsystem/PITCH ==
  note: % NOTE:  the order of the vector is:
      | %       1      2     3     4
      | %     [ U_bR,  U_fR, U_bL, U_fL ]
  Gain1 : Gain  Gain=-1
  Gain2 : Gain
  Gain3 : Gain  Gain=-1
  Gain8 : Gain
  Mux : Mux
  Sine Wave : Sin  Amplitude=m_AMP  Frequency=2*pi*f_hz_modal  SampleTime=0
      settings: AttributesFormatString=|
      | Amp =%<Amplitude>
      | w_radpsec = %<Frequency>
  Out1 : Outport
  wires:
  Gain8/1 -> Mux/1  "U_bR"
  Gain1/1 -> Mux/2  "U_fR"
  Gain2/1 -> Mux/3  "U_bL"
  Gain3/1 -> Mux/4  "U_fL"
  Sine Wave/1 -> Gain8/1, Gain1/1, Gain2/1, Gain3/1
  Mux/1 -> Out1/1

== system bh_SIM_7dof_car_MODAL_EXCITE/ROAD_SYS_MODAL/Variant Subsystem/ROLL ==
  note: % NOTE:  the order of the vector is:
      | %       1      2     3     4
      | %     [ U_bR,  U_fR, U_bL, U_fL ]
  Gain1 : Gain
  Gain2 : Gain  Gain=-1
  Gain3 : Gain  Gain=-1
  Gain8 : Gain
  Mux : Mux
  Sine Wave : Sin  Amplitude=m_AMP  Frequency=2*pi*f_hz_modal  SampleTime=0
      settings: AttributesFormatString=|
      | Amp =%<Amplitude>
      | w_radpsec = %<Frequency>
  Out1 : Outport
  wires:
  Gain8/1 -> Mux/1  "U_bR"
  Gain1/1 -> Mux/2  "U_fR"
  Gain2/1 -> Mux/3  "U_bL"
  Gain3/1 -> Mux/4  "U_fL"
  Sine Wave/1 -> Gain8/1, Gain1/1, Gain2/1, Gain3/1
  Mux/1 -> Out1/1

== system bh_SIM_7dof_car_MODAL_EXCITE/ROAD_SYS_MODAL/Variant Subsystem/SINE ==
  note: % NOTE:  the order of the vector is:
      | %       1      2     3     4
      | %     [ U_bR,  U_fR, U_bL, U_fL ]
  Gain{1..3,8} (4 alike) : Gain
  Mux : Mux
  Sine Wave : Sin  Amplitude=m_AMP  Frequency=2*pi*f_hz  SampleTime=0
      settings: AttributesFormatString=|
      | Amp =%<Amplitude>
      | w_radpsec = %<Frequency>
  Out1 : Outport
  wires:
  Gain8/1 -> Mux/1  "U_bR"
  Gain1/1 -> Mux/2  "U_fR"
  Gain2/1 -> Mux/3  "U_bL"
  Gain3/1 -> Mux/4  "U_fL"
  Sine Wave/1 -> Gain8/1, Gain1/1, Gain2/1, Gain3/1
  Mux/1 -> Out1/1

== system bh_SIM_7dof_car_MODAL_EXCITE/ROAD_SYS_MODAL/Variant Subsystem/SINE_BACK_IN ==
  note: % NOTE:  the order of the vector is:
      | %       1      2     3     4
      | %     [ U_bR,  U_fR, U_bL, U_fL ]
  Gain{1..3,8} (4 alike) : Gain
  Mux : Mux
  Sine Wave : Sin  Amplitude=m_AMP  Frequency=2*pi*f_hz  SampleTime=0
      settings: AttributesFormatString=|
      | Amp =%<Amplitude>
      | w_radpsec = %<Frequency>
  Out1 : Outport
  wires:
  Gain8/1 -> Mux/1  "U_bR"
  Gain1/1 -> Mux/2  "U_fR"
  Gain2/1 -> Mux/3  "U_bL"
  Gain3/1 -> Mux/4  "U_fL"
  Sine Wave/1 -> Gain8/1, Gain1/1, Gain2/1, Gain3/1
  Mux/1 -> Out1/1

== system bh_SIM_7dof_car_MODAL_EXCITE/ROAD_SYS_MODAL/Variant Subsystem/SINE_BACK_OUT ==
  note: % NOTE:  the order of the vector is:
      | %       1      2     3     4
      | %     [ U_bR,  U_fR, U_bL, U_fL ]
  Gain1 : Gain
  Gain2 : Gain  Gain=-1
  Gain3 : Gain
  Gain8 : Gain
  Mux : Mux
  Sine Wave : Sin  Amplitude=m_AMP  Frequency=2*pi*f_hz  SampleTime=0
      settings: AttributesFormatString=|
      | Amp =%<Amplitude>
      | w_radpsec = %<Frequency>
  Out1 : Outport
  wires:
  Gain8/1 -> Mux/1  "U_bR"
  Gain1/1 -> Mux/2  "U_fR"
  Gain2/1 -> Mux/3  "U_bL"
  Gain3/1 -> Mux/4  "U_fL"
  Sine Wave/1 -> Gain8/1, Gain1/1, Gain2/1, Gain3/1
  Mux/1 -> Out1/1

== system bh_SIM_7dof_car_MODAL_EXCITE/ROAD_SYS_MODAL/Variant Subsystem/SINE_FRONT_IN ==
  note: % NOTE:  the order of the vector is:
      | %       1      2     3     4
      | %     [ U_bR,  U_fR, U_bL, U_fL ]
  Gain{1..3,8} (4 alike) : Gain
  Mux : Mux
  Sine Wave : Sin  Amplitude=m_AMP  Frequency=2*pi*f_hz  SampleTime=0
      settings: AttributesFormatString=|
      | Amp =%<Amplitude>
      | w_radpsec = %<Frequency>
  Out1 : Outport
  wires:
  Gain8/1 -> Mux/1  "U_bR"
  Gain1/1 -> Mux/2  "U_fR"
  Gain2/1 -> Mux/3  "U_bL"
  Gain3/1 -> Mux/4  "U_fL"
  Sine Wave/1 -> Gain8/1, Gain1/1, Gain2/1, Gain3/1
  Mux/1 -> Out1/1

== system bh_SIM_7dof_car_MODAL_EXCITE/ROAD_SYS_MODAL/Variant Subsystem/SINE_FRONT_OUT ==
  note: % NOTE:  the order of the vector is:
      | %       1      2     3     4
      | %     [ U_bR,  U_fR, U_bL, U_fL ]
  Gain1 : Gain  Gain=-1
  Gain2 : Gain
  Gain3 : Gain
  Gain8 : Gain
  Mux : Mux
  Sine Wave : Sin  Amplitude=m_AMP  Frequency=2*pi*f_hz  SampleTime=0
      settings: AttributesFormatString=|
      | Amp =%<Amplitude>
      | w_radpsec = %<Frequency>
  Out1 : Outport
  wires:
  Gain8/1 -> Mux/1  "U_bR"
  Gain1/1 -> Mux/2  "U_fR"
  Gain2/1 -> Mux/3  "U_bL"
  Gain3/1 -> Mux/4  "U_fL"
  Sine Wave/1 -> Gain8/1, Gain1/1, Gain2/1, Gain3/1
  Mux/1 -> Out1/1

== system bh_SIM_7dof_car_MODAL_EXCITE/ROAD_SYS_MODAL/Variant Subsystem/SINE_PITCH ==
  note: % NOTE:  the order of the vector is:
      | %       1      2     3     4
      | %     [ U_bR,  U_fR, U_bL, U_fL ]
  Gain1 : Gain  Gain=-1
  Gain2 : Gain
  Gain3 : Gain  Gain=-1
  Gain8 : Gain
  Mux : Mux
  Sine Wave : Sin  Amplitude=m_AMP  Frequency=2*pi*f_hz  SampleTime=0
      settings: AttributesFormatString=|
      | Amp =%<Amplitude>
      | w_radpsec = %<Frequency>
  Out1 : Outport
  wires:
  Gain8/1 -> Mux/1  "U_bR"
  Gain1/1 -> Mux/2  "U_fR"
  Gain2/1 -> Mux/3  "U_bL"
  Gain3/1 -> Mux/4  "U_fL"
  Sine Wave/1 -> Gain8/1, Gain1/1, Gain2/1, Gain3/1
  Mux/1 -> Out1/1

== system bh_SIM_7dof_car_MODAL_EXCITE/ROAD_SYS_MODAL/Variant Subsystem/SINE_ROLL ==
  note: % NOTE:  the order of the vector is:
      | %       1      2     3     4
      | %     [ U_bR,  U_fR, U_bL, U_fL ]
  Gain1 : Gain
  Gain2 : Gain  Gain=-1
  Gain3 : Gain  Gain=-1
  Gain8 : Gain
  Mux : Mux
  Sine Wave : Sin  Amplitude=m_AMP  Frequency=2*pi*f_hz  SampleTime=0
      settings: AttributesFormatString=|
      | Amp =%<Amplitude>
      | w_radpsec = %<Frequency>
  Out1 : Outport
  wires:
  Gain8/1 -> Mux/1  "U_bR"
  Gain1/1 -> Mux/2  "U_fR"
  Gain2/1 -> Mux/3  "U_bL"
  Gain3/1 -> Mux/4  "U_fL"
  Sine Wave/1 -> Gain8/1, Gain1/1, Gain2/1, Gain3/1
  Mux/1 -> Out1/1
